simulink model "flexible_comp"  (R2017a)
settings: Solver=VariableStepAuto  StartTime=0.0  StopTime=20  RelTol=1e-3
values from neighbouring files (symbols this model uses):
  Amplitude = 0.2    [flexible_main.m]
  dead_zone = 0.25    [flexible_main.m]
  Frequency = 0.1    [flexible_main.m]
  Kdd = 0    [flexible_main.m]
  Kdt = 0    [flexible_main.m]
  Kpd = 0    [flexible_main.m]
  Kpt = 15    [flexible_main.m]
  saturation = 10    [flexible_main.m]
undefined symbols (not defined in the file or in its folder): p1, p2, q1, q2, r1, r2
libraries: vrlib x4
settings Model: Creator=bobbyhodgkinson  LastModifiedBy=bobbyhodgkinson
settings DataIOCC: ReturnWorkspaceOutputs=on
settings SFSimCC: SimUseLocalCustomCode=on
settings RTWCC: RTWUseLocalCustomCode=on

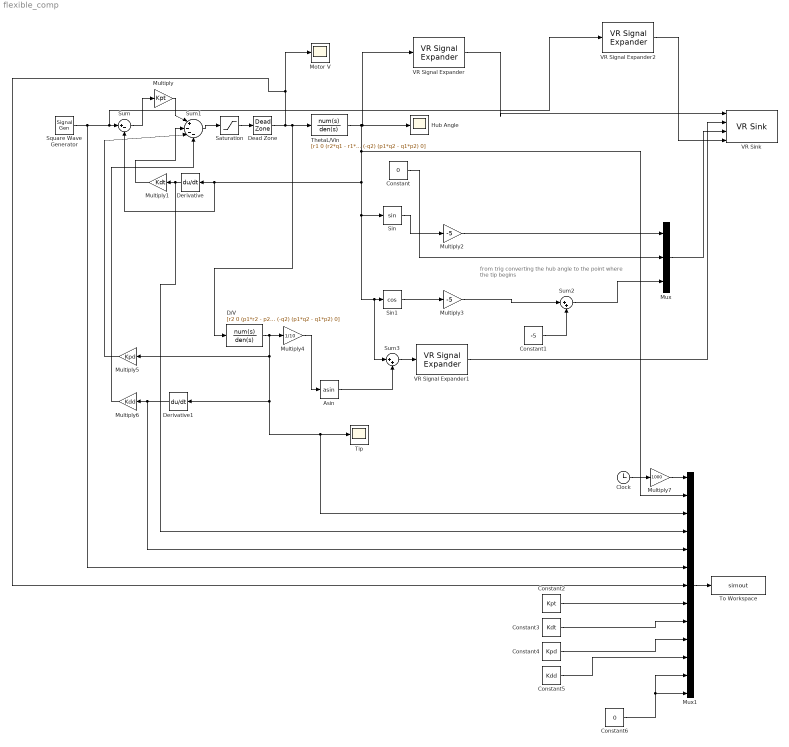
== system flexible_comp ==
  note: from trig converting the hub angle to the point where
      | the tip begins
  Asin : Trigonometry  Operator=asin
  Clock : Clock
  Constant : Constant  Value=0
  Constant1 : Constant  Value=-5
  Constant2 : Constant  Value=Kpt
  Constant3 : Constant  Value=Kdt
  Constant4 : Constant  Value=Kpd
  Constant5 : Constant  Value=Kdd
  Constant6 : Constant  Value=0
  D/V : TransferFcn  Numerator=[r2 0 (p1*r2 - p2*r1)]  Denominator=[1 (-p1) (-q2) (p1*q2 - q1*p2) 0]
  Dead Zone : DeadZone  LowerValue=-1*dead_zone  UpperValue=dead_zone  SaturateOnIntegerOverflow=on
  Derivative : Derivative  CoefficientInTFapproximation=0
  Derivative1 : Derivative  CoefficientInTFapproximation=0
  Hub Angle : Scope
  Motor V : Scope
  Multiply : Gain  Gain=Kpt
  Multiply1 : Gain  Gain=Kdt
  Multiply2 : Gain  Gain=-5
  Multiply3 : Gain  Gain=-5
  Multiply4 : Gain  Gain=1/10
  Multiply5 : Gain  Gain=Kpd
  Multiply6 : Gain  Gain=Kdd
  Multiply7 : Gain  Gain=1000
  Mux : Mux  Inputs=3
  Mux1 : Mux  Inputs=13
  Saturation : Saturate  UpperLimit=saturation  LowerLimit=-1*saturation
  Sin : Trigonometry
  Sin1 : Trigonometry  Operator=cos
  Square Wave Generator : SignalGenerator  WaveForm=square  Amplitude=Amplitude  Frequency=Frequency
  Sum : Sum  Inputs=|+-
  Sum1 : Sum  Inputs=|+---
  Sum2 : Sum  Inputs=|++
  Sum3 : Sum  Inputs=|++
  "ThetaL/Vin " : TransferFcn  Numerator=[r1 0 (r2*q1 - r1*q2)]  Denominator=[1 (-p1) (-q2) (p1*q2 - q1*p2) 0]
  Tip : Scope
  To Workspace : ToWorkspace  VariableName=simout  SaveFormat=Timeseries  SampleTime=-1
  VR Signal Expander : vrlib/VR Signal Expander  outwidth=4  outidx=[4]
      settings: SourceProductName=Simulink
  VR Signal Expander1 : vrlib/VR Signal Expander  outwidth=4  outidx=[4]
      settings: SourceProductName=Simulink
  VR Signal Expander2 : vrlib/VR Signal Expander  outwidth=4  outidx=[4]
      settings: SourceProductName=Simulink
  VR Sink : vrlib/VR Sink  InstantiateOnLoad=on  SampleTime=0.02  ViewEnable=on  RemoteChange=off  RemoteView=off  FieldsWritten=B1.rotation.4.1.1.double#Tip.rotation.4.1.1.double#Tip.translation.3.1.1.double#Ref.rotation.4.1.1.double  WorldFileName=flexible_2020.wrl  AutoView=off  VideoDimensions=[]  AllowVariableSize=off
      settings: SourceProductName=Simulink
  wires:
  Sum/1 -> Multiply/1
  Multiply/1 -> Sum1/1
  "ThetaL/Vin "/1 -> VR Signal Expander/1, Hub Angle/1, Mux1/2, Sum3/1, Sin1/1, Sin/1, Sum/2, Derivative/1
  Derivative/1 -> Mux1/4, Multiply1/1
  Multiply1/1 -> Sum1/2
  Sum1/1 -> Saturation/1
  Saturation/1 -> Dead Zone/1
  Dead Zone/1 -> Motor V/1, Mux1/7, D/V/1, "ThetaL/Vin "/1
  Constant/1 -> Mux/2
  Sin/1 -> Multiply2/1
  Sin1/1 -> Multiply3/1
  Constant1/1 -> Sum2/2
  Multiply2/1 -> Mux/1
  Multiply3/1 -> Sum2/1
  Sum2/1 -> Mux/3
  D/V/1 -> Mux1/3, Tip/1, Derivative1/1, Multiply5/1, Multiply4/1
  Multiply4/1 -> Asin/1
  Sum3/1 -> VR Signal Expander1/1
  Asin/1 -> Sum3/2
  Square Wave Generator/1 -> Mux1/6, VR Signal Expander2/1, Sum/1
  Multiply5/1 -> Sum1/3
  Derivative1/1 -> Mux1/5, Multiply6/1
  Multiply6/1 -> Sum1/4
  Mux1/1 -> To Workspace/1
  Clock/1 -> Multiply7/1
  Multiply7/1 -> Mux1/1
  Constant3/1 -> Mux1/9
  Constant5/1 -> Mux1/11
  Constant2/1 -> Mux1/8
  Constant4/1 -> Mux1/10
  Constant6/1 -> Mux1/12, Mux1/13
  VR Signal Expander/1 -> VR Sink/1
  VR Signal Expander1/1 -> VR Sink/2
  Mux/1 -> VR Sink/3
  VR Signal Expander2/1 -> VR Sink/4
